simulink model "secant"  (R2021a)
settings: Solver=FixedStepDiscrete  StartTime=0.0  StopTime=inf  FixedStep=1  RelTol=1e-3
libraries: simulink x1
settings Model: Creator=manur  LastModifiedBy=manur

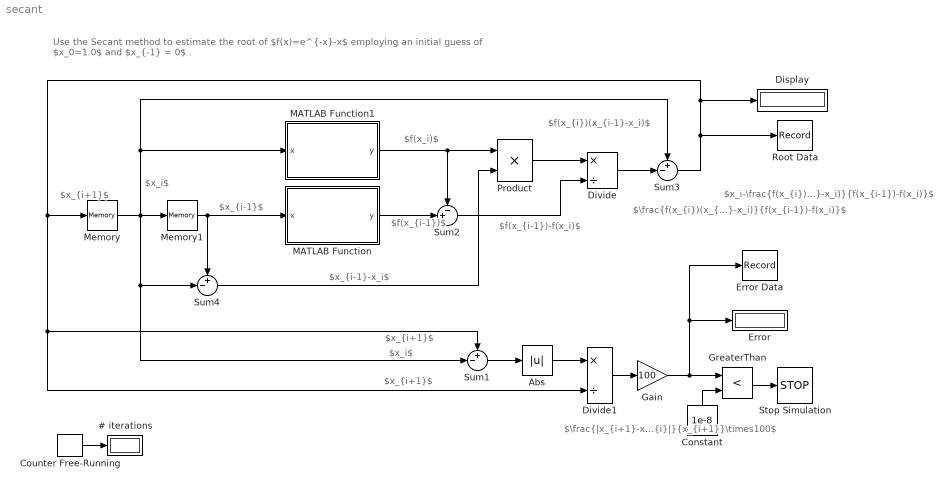
== system secant ==
  note: $x_i$
  note: $f(x_{i-1})$
  note: Use the Secant method to estimate the root of $f(x)=e^{-x}-x$ employing an initial guess of $x_0=1.0$ and $x_{-1} = 0$ .
  note: $f(x_i)$
  note: $x_{i+1}$
  note: $\frac{|x_{i+1}-x_{i}|}{x_{i+1}}\times100$
  note: $x_{i+1}$
  note: $x_i$
  note: $x_{i+1}$
  note: $x_{i-1}$
  note: $x_{i-1}-x_i$
  note: $f(x_{i-1})-f(x_i)$
  note: $f(x_{i})(x_{i-1}-x_i)$
  note: $\frac{f(x_{i})(x_{i-1}-x_i)}{f(x_{i-1})-f(x_i)}$
  note: $x_i-\frac{f(x_{i})(x_{i-1}-x_i)}{f(x_{i-1})-f(x_i)}$
  # iterations : Display
  Abs : Abs
  Constant : Constant  Value=1e-8
  Counter Free-Running : simulink/Sources/Counter Free-Running  NumBits=16  tsamp=-1
  Display : Display
  Divide : Product  Inputs=*/
  Divide1 : Product  Inputs=*/
  Error : Display
  Error Data : Record  FileSettingsInternal="{\"entries\":[{\"content\":{\"excelSettings\":{\"content\":{},\"type\":\"Streamout.ExcelSettings\"}},\"type\":\"Streamout.FileSettingStorage\",\"uuid\":\"ce780b49-f8fc-47f1-a22b-1c643ce1729d\"}],\"packageUris\":[\"http://schema.mathworks.com/mf0/streamout_blocks/R2020a\"],\"version\":\"1.0\"}"  SignalsInternal="{\"entries\":[{\"content\":{\"signals\":[{\"content\":{\"blockPath\":[\"secant/Error Data\"],\"channel\":[],\"dimensions\":[1],\"domain\":\"secant/error data\",\"lineColor\":\"#fe330a\",\"plots\":[1],\"port\":1,\"sid\":[],\"signalID\":336,\"signalName\":\"Gain\"},\"type\":\"RecordBlkView.Signal\",\"uuid\":\"27531e50-fd39-4feb-8290-fe6a89478337\"}]},\"type\":\"RecordBlkView.InputSignals\",\"uuid\":\"8fc0a6ad-9e9e-4774-b9d4-871cbd668533\"}],\"packageUris\":[\"http://schema.mathworks.com/mf0/streamout_blocks/R2020a\"],\"version\":\"1.0\"}"  VisualizationBindings="{\"sparklinesplugin\":{\"info\":[{\"bindingParametersList\":[],\"subplotID\":1}]}}"
  Gain : Gain  Gain=100
  GreaterThan : RelationalOperator  Operator=<  OutDataTypeStr=boolean  RndMeth=Simplest
  MATLAB Function : MATLAB Function  TreatAsAtomicUnit=on
  MATLAB Function1 : MATLAB Function  TreatAsAtomicUnit=on
  Memory : Memory  InitialCondition=1
  Memory1 : Memory
  Product : Product
  Root Data : Record  FileSettingsInternal="{\"entries\":[{\"content\":{\"excelSettings\":{\"content\":{},\"type\":\"Streamout.ExcelSettings\"}},\"type\":\"Streamout.FileSettingStorage\",\"uuid\":\"bc5a132c-1ffa-4a8c-89b3-128a7b384f57\"}],\"packageUris\":[\"http://schema.mathworks.com/mf0/streamout_blocks/R2020a\"],\"version\":\"1.0\"}"  SignalsInternal="{\"entries\":[{\"content\":{\"signals\":[{\"content\":{\"blockPath\":[\"secant/Root Data\"],\"channel\":[],\"dimensions\":[1],\"domain\":\"secant/root data\",\"lineColor\":\"#b746ff\",\"plots\":[1],\"port\":1,\"sid\":[],\"signalID\":331,\"signalName\":\"Sum3\"},\"type\":\"RecordBlkView.Signal\",\"uuid\":\"a6dccb1b-d194-4500-9bdc-5b1c450104aa\"}]},\"type\":\"RecordBlkView.InputSignals\",\"uuid\":\"f65f23b5-17ad-494b-b8e5-e99a9e1211db\"}],\"packageUris\":[\"http://schema.mathworks.com/mf0/streamout_blocks/R2020a\"],\"version\":\"1.0\"}"  VisualizationBindings="{\"sparklinesplugin\":{\"info\":[{\"bindingParametersList\":[],\"subplotID\":1}]}}"
  Stop Simulation : Stop
  Sum1 : Sum  Inputs=+-|
  Sum2 : Sum  Inputs=-+|
  Sum3 : Sum  Inputs=+-|
  Sum4 : Sum  Inputs=+-|
  wires:
  Memory/1 -> Sum1/2, Sum4/2, MATLAB Function1/1(x), Sum3/1, Memory1/1
  Sum1/1 -> Abs/1
  Divide1/1 -> Gain/1
  Abs/1 -> Divide1/1
  Constant/1 -> GreaterThan/2
  GreaterThan/1 -> Stop Simulation/1
  Gain/1 -> GreaterThan/1, Error/1, Error Data/1
  Counter Free-Running/1 -> # iterations/1
  Memory1/1 -> MATLAB Function/1(x), Sum4/1
  Sum4/1 -> Product/2
  MATLAB Function1/1(y) -> Sum2/1, Product/1
  MATLAB Function/1(y) -> Sum2/2
  Product/1 -> Divide/1
  Sum2/1 -> Divide/2
  Divide/1 -> Sum3/2
  Sum3/1 -> Root Data/1, Display/1, Sum1/1, Divide1/2, Memory/1

== matlab function secant/MATLAB Function ==
  data: x input; y output
function y = f(x)

y = exp(-x)-x;

== matlab function secant/MATLAB Function1 ==
  data: x input; y output
function y = f(x)

y = exp(-x)-x;
